simulink model "pressure_check"  (R2025a)
settings: Solver=VariableStepAuto  StartTime=0.0  StopTime=inf  RelTol=1e-3
undefined symbols (not defined in the file or in its folder): National_Instruments, PCI
libraries: sldrtlib x13
settings Model: Creator=dperera  LastModifiedBy=dperera

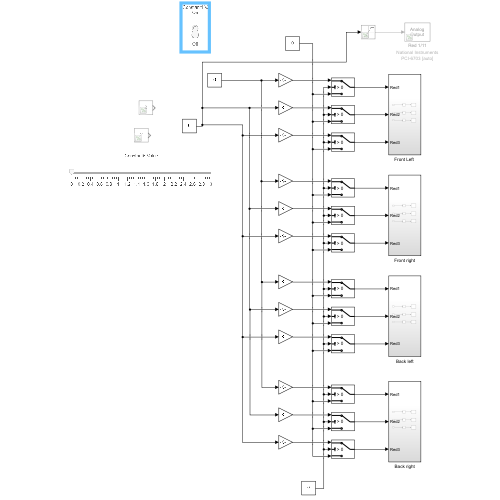
[thumbnail: Simulink's stored preview of the top-level diagram]
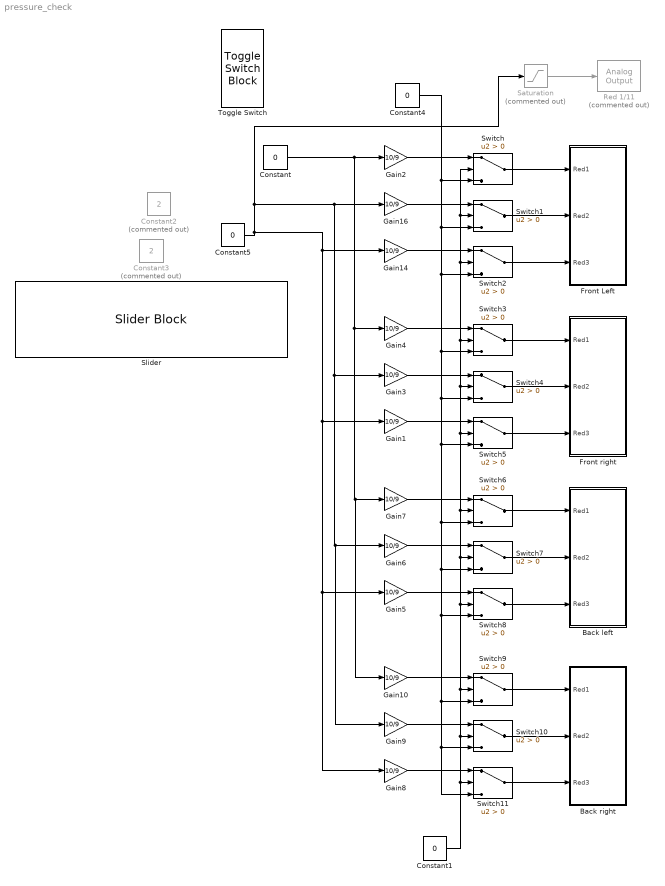
== system pressure_check ==
  Back left : Subsystem
  Back right : Subsystem
  Constant{,1,4..5} (4 alike) : Constant  Value=0
  Constant2 : Constant  Commented=on  Value=2
  Constant3 : Constant  Commented=on  Value=2
  "Front Left " : Subsystem
  Front right : Subsystem
  Gain{1..10,14,16} (12 alike) : Gain  Gain=10/9
  Red 1/11 : sldrtlib/Analog Output  Commented=on  SampleTime=0.01  MaxMissedTicks=inf  ShowMissedTicks=off  YieldWhenWaiting=on  DrvName=National_Instruments/PCI-6703  DrvAddress=4294967295  DrvOptions=0  Channels=12  RangeMode=1  VoltRange=1  InitialValue=0  FinalValue=0
      settings: AttributesFormatString=National Instruments\nPCI-6703 [auto]
  Saturation : Saturate  Commented=on  UpperLimit=7  LowerLimit=0
  Slider : SliderBlock  ScaleMax=3
  Switch{,1..11} (12 alike) : Switch  Criteria=u2 > Threshold  SaturateOnIntegerOverflow=off  InputSameDT=off
  Toggle Switch : ToggleSwitchBlock
  wires:
  Switch/1 -> "Front Left "/1(Red1)
  Constant4/1 -> Switch3/3, Switch4/3, Switch5/3, Switch6/3, Switch8/3, Switch9/3, Switch10/3, Switch11/3, Switch7/3, Switch2/3, Switch1/3, Switch/3
  Switch1/1 -> "Front Left "/2(Red2)
  Gain2/1 -> Switch/1
  Constant1/1 -> Switch11/2, Switch9/2, Switch5/2, Switch4/2, Switch3/2, Switch2/2, Switch1/2, Switch/2, Switch6/2, Switch7/2, Switch8/2, Switch10/2
  Switch2/1 -> "Front Left "/3(Red3)
  Gain14/1 -> Switch2/1
  Gain16/1 -> Switch1/1
  Switch5/1 -> Front right/3(Red3)
  Switch4/1 -> Front right/2(Red2)
  Switch3/1 -> Front right/1(Red1)
  Gain4/1 -> Switch3/1
  Gain3/1 -> Switch4/1
  Gain1/1 -> Switch5/1
  Gain5/1 -> Switch8/1
  Gain6/1 -> Switch7/1
  Gain7/1 -> Switch6/1
  Switch6/1 -> Back left/1(Red1)
  Switch7/1 -> Back left/2(Red2)
  Switch8/1 -> Back left/3(Red3)
  Switch10/1 -> Back right/2(Red2)
  Switch9/1 -> Back right/1(Red1)
  Gain10/1 -> Switch9/1
  Gain9/1 -> Switch10/1
  Switch11/1 -> Back right/3(Red3)
  Gain8/1 -> Switch11/1
  Constant/1 -> Gain10/1, Gain7/1, Gain4/1, Gain2/1
  Constant5/1 -> Gain8/1, Gain5/1, Gain1/1, Gain14/1, Gain3/1, Gain9/1, Gain6/1, Gain16/1, Saturation/1
  Saturation/1 -> Red 1/11/1

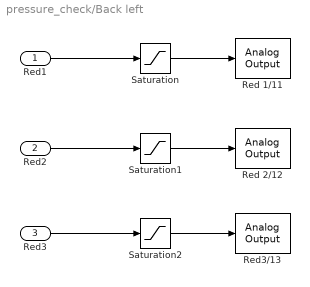
== system pressure_check/Back left ==
  Red1 : Inport
  Red2 : Inport  Port=2
  Red3 : Inport  Port=3
  Red 1/11 : sldrtlib/Analog Output  SampleTime=0.01  MaxMissedTicks=inf  ShowMissedTicks=off  YieldWhenWaiting=on  DrvName=National_Instruments/PCI-6703  DrvAddress=4294967295  DrvOptions=0  Channels=8  RangeMode=1  VoltRange=1  InitialValue=[]  FinalValue=[]
      settings: AttributesFormatString=National Instruments\nPCI-6703 [auto]
  Red 2/12 : sldrtlib/Analog Output  SampleTime=0.01  MaxMissedTicks=inf  ShowMissedTicks=off  YieldWhenWaiting=on  DrvName=National_Instruments/PCI-6703  DrvAddress=4294967295  DrvOptions=0  Channels=9  RangeMode=1  VoltRange=1  InitialValue=[]  FinalValue=[]
      settings: AttributesFormatString=National Instruments\nPCI-6703 [auto]
  Red3/13 : sldrtlib/Analog Output  SampleTime=0.01  MaxMissedTicks=inf  ShowMissedTicks=off  YieldWhenWaiting=on  DrvName=National_Instruments/PCI-6703  DrvAddress=4294967295  DrvOptions=0  Channels=10  RangeMode=1  VoltRange=1  InitialValue=[]  FinalValue=[]
      settings: AttributesFormatString=National Instruments\nPCI-6703 [auto]
  Saturation : Saturate  UpperLimit=7  LowerLimit=0
  Saturation1 : Saturate  UpperLimit=7  LowerLimit=0
  Saturation2 : Saturate  UpperLimit=7  LowerLimit=0
  wires:
  Red1/1 -> Saturation/1
  Saturation/1 -> Red 1/11/1
  Saturation1/1 -> Red 2/12/1
  Saturation2/1 -> Red3/13/1
  Red2/1 -> Saturation1/1
  Red3/1 -> Saturation2/1

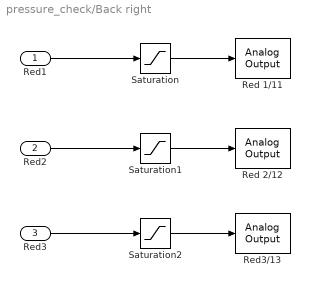
== system pressure_check/Back right ==
  Red1 : Inport
  Red2 : Inport  Port=2
  Red3 : Inport  Port=3
  Red 1/11 : sldrtlib/Analog Output  SampleTime=0.01  MaxMissedTicks=inf  ShowMissedTicks=off  YieldWhenWaiting=on  DrvName=National_Instruments/PCI-6703  DrvAddress=4294967295  DrvOptions=0  Channels=11  RangeMode=1  VoltRange=1  InitialValue=[]  FinalValue=[]
      settings: AttributesFormatString=National Instruments\nPCI-6703 [auto]
  Red 2/12 : sldrtlib/Analog Output  SampleTime=0.01  MaxMissedTicks=inf  ShowMissedTicks=off  YieldWhenWaiting=on  DrvName=National_Instruments/PCI-6703  DrvAddress=4294967295  DrvOptions=0  Channels=12  RangeMode=1  VoltRange=1  InitialValue=0  FinalValue=0
      settings: AttributesFormatString=National Instruments\nPCI-6703 [auto]
  Red3/13 : sldrtlib/Analog Output  SampleTime=0.01  MaxMissedTicks=inf  ShowMissedTicks=off  YieldWhenWaiting=on  DrvName=National_Instruments/PCI-6703  DrvAddress=4294967295  DrvOptions=0  Channels=13  RangeMode=1  VoltRange=1  InitialValue=[]  FinalValue=[]
      settings: AttributesFormatString=National Instruments\nPCI-6703 [auto]
  Saturation : Saturate  UpperLimit=7  LowerLimit=0
  Saturation1 : Saturate  UpperLimit=7  LowerLimit=0
  Saturation2 : Saturate  UpperLimit=7  LowerLimit=0
  wires:
  Red3/1 -> Saturation2/1
  Red2/1 -> Saturation1/1
  Saturation2/1 -> Red3/13/1
  Saturation1/1 -> Red 2/12/1
  Saturation/1 -> Red 1/11/1
  Red1/1 -> Saturation/1

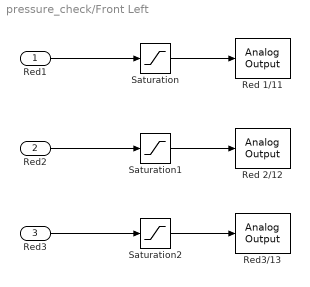
== system pressure_check/Front Left  ==
  Red1 : Inport
  Red2 : Inport  Port=2
  Red3 : Inport  Port=3
  Red 1/11 : sldrtlib/Analog Output  SampleTime=0.01  MaxMissedTicks=inf  ShowMissedTicks=off  YieldWhenWaiting=on  DrvName=National_Instruments/PCI-6703  DrvAddress=4294967295  DrvOptions=0  Channels=1  RangeMode=1  VoltRange=1  InitialValue=0  FinalValue=0
      settings: AttributesFormatString=National Instruments\nPCI-6703 [auto]
  Red 2/12 : sldrtlib/Analog Output  SampleTime=0.01  MaxMissedTicks=inf  ShowMissedTicks=off  YieldWhenWaiting=on  DrvName=National_Instruments/PCI-6703  DrvAddress=4294967295  DrvOptions=0  Channels=2  RangeMode=1  VoltRange=1  InitialValue=0  FinalValue=0
      settings: AttributesFormatString=National Instruments\nPCI-6703 [auto]
  Red3/13 : sldrtlib/Analog Output  SampleTime=0.01  MaxMissedTicks=inf  ShowMissedTicks=off  YieldWhenWaiting=on  DrvName=National_Instruments/PCI-6703  DrvAddress=4294967295  DrvOptions=0  Channels=3  RangeMode=1  VoltRange=1  InitialValue=0  FinalValue=0
      settings: AttributesFormatString=National Instruments\nPCI-6703 [auto]
  Saturation : Saturate  UpperLimit=7  LowerLimit=0
  Saturation1 : Saturate  UpperLimit=7  LowerLimit=0
  Saturation2 : Saturate  UpperLimit=7  LowerLimit=0
  wires:
  Red1/1 -> Saturation/1
  Saturation/1 -> Red 1/11/1
  Saturation1/1 -> Red 2/12/1
  Saturation2/1 -> Red3/13/1
  Red2/1 -> Saturation1/1
  Red3/1 -> Saturation2/1

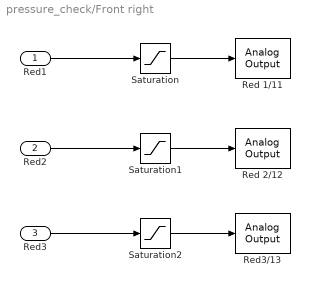
== system pressure_check/Front right ==
  Red1 : Inport
  Red2 : Inport  Port=2
  Red3 : Inport  Port=3
  Red 1/11 : sldrtlib/Analog Output  SampleTime=0.01  MaxMissedTicks=inf  ShowMissedTicks=off  YieldWhenWaiting=on  DrvName=National_Instruments/PCI-6703  DrvAddress=4294967295  DrvOptions=0  Channels=5  RangeMode=1  VoltRange=1  InitialValue=0  FinalValue=0
      settings: AttributesFormatString=National Instruments\nPCI-6703 [auto]
  Red 2/12 : sldrtlib/Analog Output  SampleTime=0.01  MaxMissedTicks=inf  ShowMissedTicks=off  YieldWhenWaiting=on  DrvName=National_Instruments/PCI-6703  DrvAddress=4294967295  DrvOptions=0  Channels=6  RangeMode=1  VoltRange=1  InitialValue=[]  FinalValue=[]
      settings: AttributesFormatString=National Instruments\nPCI-6703 [auto]
  Red3/13 : sldrtlib/Analog Output  SampleTime=0.01  MaxMissedTicks=inf  ShowMissedTicks=off  YieldWhenWaiting=on  DrvName=National_Instruments/PCI-6703  DrvAddress=4294967295  DrvOptions=0  Channels=7  RangeMode=1  VoltRange=1  InitialValue=[]  FinalValue=[]
      settings: AttributesFormatString=National Instruments\nPCI-6703 [auto]
  Saturation : Saturate  UpperLimit=7  LowerLimit=0
  Saturation1 : Saturate  UpperLimit=7  LowerLimit=0
  Saturation2 : Saturate  UpperLimit=7  LowerLimit=0
  wires:
  Red3/1 -> Saturation2/1
  Red2/1 -> Saturation1/1
  Saturation2/1 -> Red3/13/1
  Saturation1/1 -> Red 2/12/1
  Saturation/1 -> Red 1/11/1
  Red1/1 -> Saturation/1
